simulink model "mcb_hall_foc_host"  (R2021a)
settings: Solver=FixedStepDiscrete  StartTime=0.0  StopTime=inf  RelTol=1e-3  EnableMultiTasking=on
values from neighbouring files (symbols this model uses):
  PU_System = mcb_SetPUSystem(pmsm,inverter)    [mcb_pmsm_foc_hall_MCSPTE1AK144_data.m]
  Ts_uart = 0.01    [mcb_pmsm_foc_hall_MCSPTE1AK144_data.m]
libraries: mcbhostblockslib x3, simulink x3
settings Model: Creator=The MathWorks, Inc.  LastModifiedBy=Prasad Hegde
settings SolverCC: AlgebraicLoopSolver=TrustRegion
settings DataIOCC: LimitDataPoints=on  SaveFormat=Array  ReturnWorkspaceOutputs=off
settings OptimizationCC: LifeSpan=1  EfficientTunableParamExpr=on
settings DebuggingCC: MergeDetectMultiDrivingBlocksExec=none  SolverPrmCheckMsg=warning  ParameterPrecisionLossMsg=none  AllowSymbolicDim=off  PregeneratedLibrarySubsystemCodeDiagnostic=none  SFUnexpectedBacktrackingDiag=warning  SFNoUnconditionalDefaultTransitionDiag=warning  SFExecutionAtInitializationDiag=none  SFMachineParentedDataDiag=warning  ArithmeticOperatorsInVariantConditions=warning
settings HardwareCC: ProdBitPerPointer=32  ProdLargestAtomicFloat=None  ProdIntDivRoundTo=Undefined  ProdEndianess=Unspecified  ProdWordSize=32  ProdHWDeviceType=32-bit Generic
settings ModelReferenceCC: PropagateSignalLabelsOutOfModel=off
settings SFSimCC: SimUseLocalCustomCode=off  MATLABDynamicMemAlloc=off
settings RTWCC: Description=Real-Time Workshop Embedded Coder  SystemTargetFile=ert.tlc  TemplateMakefile=ert_default_tmf  GenerateReport=on  RTWUseLocalCustomCode=off  IncludeHyperlinkInReport=on  LaunchReport=on  GenerateTraceInfo=on  GenerateTraceReport=on  GenerateTraceReportSl=on  GenerateTraceReportSf=on  GenerateTraceReportEml=on
settings CodeAppCC: IgnoreCustomStorageClasses=off  StateflowObjectComments=on  InternalIdentifier=Classic
settings ERTTargetCC: MultiwordLength=2048  GenerateSampleERTMain=on  ERTCustomFileTemplate=example_file_process.tlc  ConvertIfToSwitch=off  SuppressUnreachableDefaultCases=off
settings ConfigComp: CovMetricSettings=dw  CovSaveCumulativeToWorkspaceVar=on  CovSaveSingleToWorkspaceVar=on  CovExternalEMLEnable=off  CovSFcnEnable=off

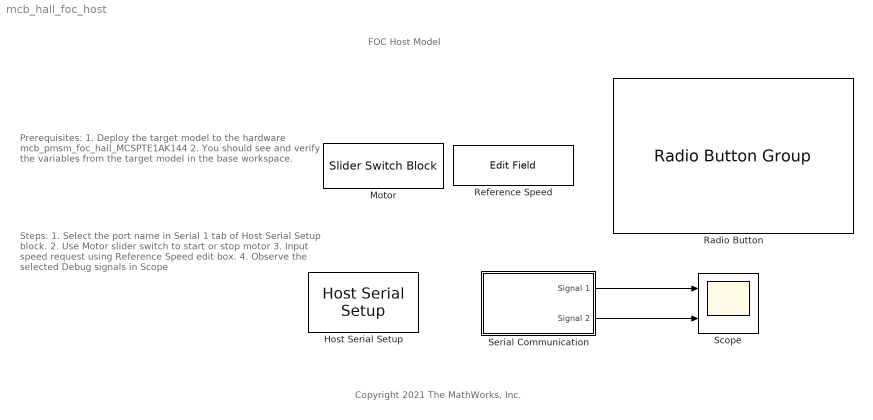
== system mcb_hall_foc_host ==
  note: FOC Host Model
  note: Steps:
      | 1. Select the port name in Serial 1 tab of
      | Host Serial Setup block.
      | 2. Use Motor slider switch to start or stop motor
      | 3. Input speed request using Reference Speed
      | edit box.
      | 4. Observe the selected Debug signals in Scope
  note: Prerequisites:
      | 1. Deploy the target model to the hardware
      | mcb_pmsm_foc_hall_MCSPTE1AK144
      |
      | 2. You should see and verify the variables
      | from the target model in the base
      | workspace.
  note: Copyright 2021 The MathWorks, Inc.
  Host Serial Setup : mcbhostblockslib/Host Serial Setup  Priority=-99  comPortSer1='Please_select_a_port'  baudRateA=256000  charLenA=8  stopBitA=1  parityA=none  timeoutA=2  ByteOrderA=LittleEndian  comPortSer2='Please_select_a_port'  baudRateB=115200  charLenB=8  stopBitB=1  parityB=none  timeoutB=1.0  ByteOrderB=LittleEndian  comPortSer3='Please_select_a_port'  baudRateC=115200  charLenC=8  stopBitC=1  parityC=none  timeoutC=1.0  ByteOrderC=LittleEndian  comPortSer4='Please_select_a_port'  baudRateD=115200  charLenD=8  stopBitD=1  parityD=none  timeoutD=1.0  ByteOrderD=LittleEndian
      settings: SourceProductBaseCode=MT
  Motor : SliderSwitchBlock  LabelPosition=Hide
      settings: Values={{'Stop', 'Start'}, [0 1]}
  Radio Button : RadioButtonGroup  LabelPosition=Hide  SelectedLabel=Speed_ref & Speed_feedback  ButtonGroupName=Debug signals
      settings: Values={{'Speed_ref & Speed_feedback', 'Id_ref & Id_feedback', 'Iq_ref & Iq_feedback', 'Ia & Ib', 'Ia & Position'}, [1 2 3 4 5]}
  Reference Speed : EditField  LabelPosition=Hide  ShowInitialText=on  Alignment=Center
  Scope : Scope  NumInputPorts=2
  Serial Communication : Subsystem
  wires:
  Serial Communication/1(Signal 1) -> Scope/1
  Serial Communication/2(Signal 2) -> Scope/2

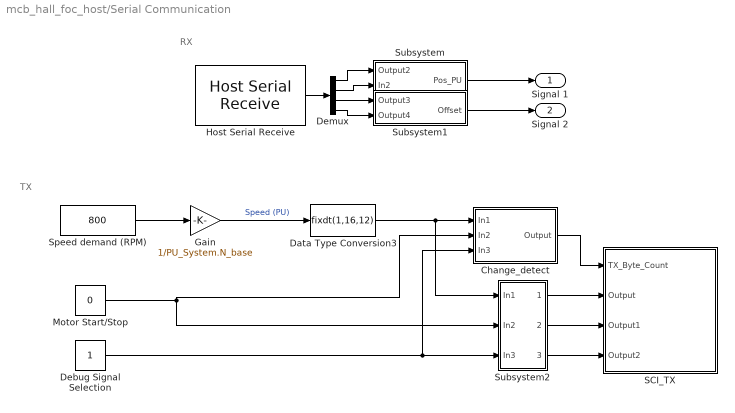
== system mcb_hall_foc_host/Serial Communication ==
  note: RX
  note: TX
  Change_detect : Subsystem
  Data Type Conversion3 : DataTypeConversion  OutDataTypeStr=fixdt(1,16,12)  RndMeth=Simplest
  Debug Signal Selection : Constant  OutDataTypeStr=Inherit: Inherit via back propagation
  Demux : Demux
  Gain : Gain  Gain=1/PU_System.N_base  RndMeth=Simplest  OutDataTypeStr=Inherit: Same as input
  Host Serial Receive : mcbhostblockslib/Host Serial Receive  serialCon=Serial 1  dataHead='S'  dataTail='E'  dataType=uint8  dataDim=4  initValue=5  errOption=Output custom value  errValue=15  sampleTime=Ts_uart  outputStatus=off  blockingMode=on
      settings: SourceProductBaseCode=MT
  Motor Start/Stop : Constant  Value=0  OutDataTypeStr=Inherit: Inherit via back propagation
  SCI_TX : Subsystem  TreatAsAtomicUnit=on
  Speed demand (RPM) : Constant  Value=800  VectorParams1D=off  OutDataTypeStr=single  SampleTime=Ts_uart * 100
  Subsystem : Subsystem
  Subsystem1 : Subsystem
  Subsystem2 : Subsystem
  Signal 1 : Outport
  Signal 2 : Outport  Port=2
  wires:
  Motor Start/Stop/1 -> Change_detect/2(In2), Subsystem2/2(In2)
  Subsystem/1(Pos_PU) -> Signal 1/1
  Subsystem1/1(Offset) -> Signal 2/1
  Speed demand (RPM)/1 -> Gain/1
  Gain/1 -> Data Type Conversion3/1  "Speed (PU)"
  Host Serial Receive/1 -> Demux/1
  Demux/2 -> Subsystem/2(In2)
  Demux/1 -> Subsystem/1(Output2)
  Demux/3 -> Subsystem1/1(Output3)
  Demux/4 -> Subsystem1/2(Output4)
  Debug Signal Selection/1 -> Subsystem2/3(In3), Change_detect/3(In3)
  Subsystem2/1(Output) -> SCI_TX/2(Output)
  Subsystem2/2(Output1) -> SCI_TX/3(Output1)
  Subsystem2/3(Output2) -> SCI_TX/4(Output2)
  Change_detect/1(Output) -> SCI_TX/1(TX_Byte_Count)
  Data Type Conversion3/1 -> Change_detect/1(In1), Subsystem2/1(In1)

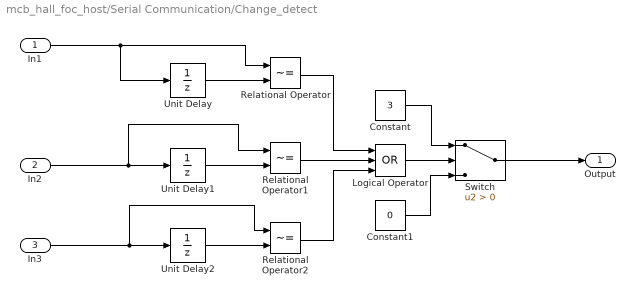
== system mcb_hall_foc_host/Serial Communication/Change_detect ==
  In1 : Inport
  In2 : Inport  Port=2
  In3 : Inport  Port=3
  Constant : Constant  Value=3  OutDataTypeStr=uint8
  Constant1 : Constant  Value=0  OutDataTypeStr=uint8
  Logical Operator : Logic  Operator=OR  Inputs=3  AllPortsSameDT=off  OutDataTypeStr=boolean
  Relational Operator : RelationalOperator  Operator=~=  OutDataTypeStr=boolean  RndMeth=Nearest
  Relational Operator1 : RelationalOperator  Operator=~=  OutDataTypeStr=boolean  RndMeth=Nearest
  Relational Operator2 : RelationalOperator  Operator=~=  OutDataTypeStr=boolean  RndMeth=Nearest
  Switch : Switch  Criteria=u2 > Threshold
  Unit Delay : UnitDelay  InitialCondition=0.5  SampleTime=-1  HasFrameUpgradeWarning=on
  Unit Delay1 : UnitDelay  SampleTime=-1  HasFrameUpgradeWarning=on
  Unit Delay2 : UnitDelay  SampleTime=-1  HasFrameUpgradeWarning=on
  Output : Outport
  wires:
  In2/1 -> Relational Operator1/1, Unit Delay1/1
  Unit Delay1/1 -> Relational Operator1/2
  Relational Operator1/1 -> Logical Operator/2
  Unit Delay/1 -> Relational Operator/2
  In1/1 -> Relational Operator/1, Unit Delay/1
  Relational Operator/1 -> Logical Operator/1
  Relational Operator2/1 -> Logical Operator/3
  Unit Delay2/1 -> Relational Operator2/2
  In3/1 -> Relational Operator2/1, Unit Delay2/1
  Switch/1 -> Output/1
  Logical Operator/1 -> Switch/2
  Constant/1 -> Switch/1
  Constant1/1 -> Switch/3

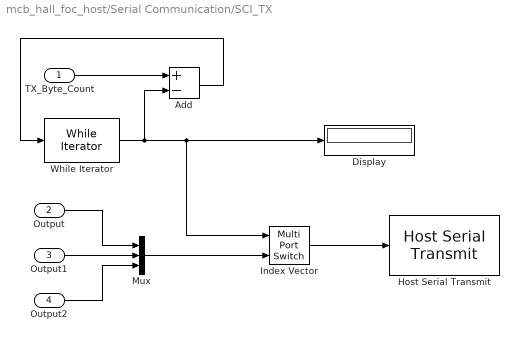
== system mcb_hall_foc_host/Serial Communication/SCI_TX ==
  TX_Byte_Count : Inport
  Output : Inport  Port=2
  Output1 : Inport  Port=3
  Output2 : Inport  Port=4
  Add : Sum  Inputs=+-  OutDataTypeStr=Inherit: Same as first input
  Display : Display
  Host Serial Transmit : mcbhostblockslib/Host Serial Transmit  serialCon=Serial 1  header=''  tail=''  enableBlockingMode=off
      settings: SourceProductBaseCode=MT
  Index Vector : MultiPortSwitch  Inputs=1
  Mux : Mux  Inputs=3
  While Iterator : WhileIterator  MaxIters=3  WhileBlockType=do-while  ShowIterationPort=on  OutputDataType=int16
  wires:
  Output/1 -> Mux/1
  Output2/1 -> Mux/3
  Output1/1 -> Mux/2
  Mux/1 -> Index Vector/2
  Index Vector/1 -> Host Serial Transmit/1
  TX_Byte_Count/1 -> Add/1
  Add/1 -> While Iterator/1
  While Iterator/1 -> Index Vector/1, Display/1, Add/2

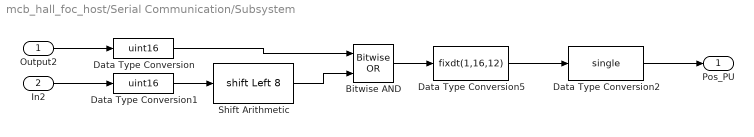
== system mcb_hall_foc_host/Serial Communication/Subsystem ==
  Output2 : Inport
  In2 : Inport  Port=2
  Bitwise AND : simulink/Logic and Bit Operations/Bitwise Operator  logicop=OR  UseBitMask=off  NumInputPorts=2  BitMask=bin2dec('11011001')  BitMaskRealWorld=Stored Integer
  Data Type Conversion : DataTypeConversion  OutDataTypeStr=uint16  RndMeth=Simplest
  Data Type Conversion1 : DataTypeConversion  OutDataTypeStr=uint16  RndMeth=Simplest
  Data Type Conversion2 : DataTypeConversion  OutDataTypeStr=single  RndMeth=Simplest
  Data Type Conversion5 : DataTypeConversion  OutDataTypeStr=fixdt(1,16,12)  ConvertRealWorld=Stored Integer (SI)  RndMeth=Simplest
  Shift Arithmetic : ArithShift  BitShiftNumber=8  BitShiftDirection=Left
  Pos_PU : Outport
  wires:
  Output2/1 -> Data Type Conversion/1
  Data Type Conversion5/1 -> Data Type Conversion2/1
  In2/1 -> Data Type Conversion1/1
  Shift Arithmetic/1 -> Bitwise AND/2
  Bitwise AND/1 -> Data Type Conversion5/1
  Data Type Conversion1/1 -> Shift Arithmetic/1
  Data Type Conversion/1 -> Bitwise AND/1
  Data Type Conversion2/1 -> Pos_PU/1

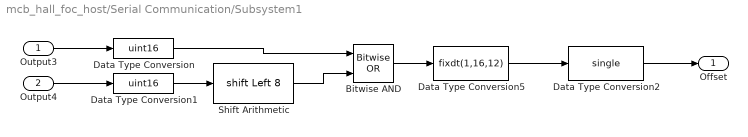
== system mcb_hall_foc_host/Serial Communication/Subsystem1 ==
  Output3 : Inport
  Output4 : Inport  Port=2
  Bitwise AND : simulink/Logic and Bit Operations/Bitwise Operator  logicop=OR  UseBitMask=off  NumInputPorts=2  BitMask=bin2dec('11011001')  BitMaskRealWorld=Stored Integer
  Data Type Conversion : DataTypeConversion  OutDataTypeStr=uint16  RndMeth=Simplest
  Data Type Conversion1 : DataTypeConversion  OutDataTypeStr=uint16  RndMeth=Simplest
  Data Type Conversion2 : DataTypeConversion  OutDataTypeStr=single  RndMeth=Simplest
  Data Type Conversion5 : DataTypeConversion  OutDataTypeStr=fixdt(1,16,12)  ConvertRealWorld=Stored Integer (SI)  RndMeth=Simplest
  Shift Arithmetic : ArithShift  BitShiftNumber=8  BitShiftDirection=Left
  Offset : Outport
  wires:
  Data Type Conversion/1 -> Bitwise AND/1
  Data Type Conversion1/1 -> Shift Arithmetic/1
  Bitwise AND/1 -> Data Type Conversion5/1
  Shift Arithmetic/1 -> Bitwise AND/2
  Output4/1 -> Data Type Conversion1/1
  Data Type Conversion5/1 -> Data Type Conversion2/1
  Output3/1 -> Data Type Conversion/1
  Data Type Conversion2/1 -> Offset/1

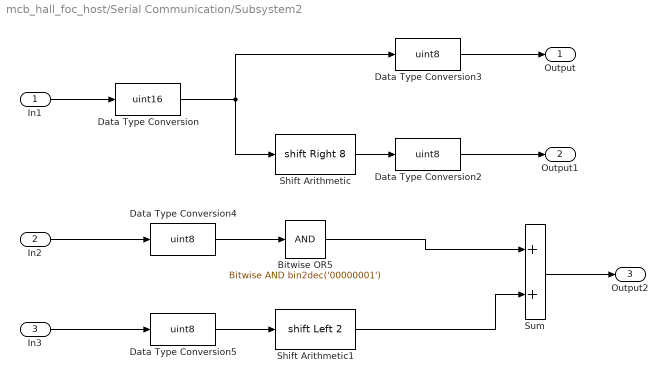
== system mcb_hall_foc_host/Serial Communication/Subsystem2 ==
  In1 : Inport
  In2 : Inport  Port=2
  In3 : Inport  Port=3
  Bitwise OR5 : simulink/Logic and Bit Operations/Bitwise Operator  logicop=AND  UseBitMask=on  BitMask=bin2dec('00000001')  BitMaskRealWorld=Stored Integer
  Data Type Conversion : DataTypeConversion  OutDataTypeStr=uint16  ConvertRealWorld=Stored Integer (SI)  RndMeth=Simplest
  Data Type Conversion{2..5} (4 alike) : DataTypeConversion  OutDataTypeStr=uint8  ConvertRealWorld=Stored Integer (SI)  RndMeth=Simplest
  Shift Arithmetic : ArithShift  BitShiftNumber=8  BitShiftDirection=Right
  Shift Arithmetic1 : ArithShift  BitShiftNumber=2  BitShiftDirection=Left
  Sum : Sum
  Output : Outport
  Output1 : Outport  Port=2
  Output2 : Outport  Port=3
  wires:
  Data Type Conversion5/1 -> Shift Arithmetic1/1
  Bitwise OR5/1 -> Sum/1
  In1/1 -> Data Type Conversion/1
  Data Type Conversion/1 -> Shift Arithmetic/1, Data Type Conversion3/1
  Shift Arithmetic1/1 -> Sum/2
  Data Type Conversion4/1 -> Bitwise OR5/1
  Sum/1 -> Output2/1
  Shift Arithmetic/1 -> Data Type Conversion2/1
  In2/1 -> Data Type Conversion4/1
  In3/1 -> Data Type Conversion5/1
  Data Type Conversion2/1 -> Output1/1
  Data Type Conversion3/1 -> Output/1
